simulink subsystem "NAV_GYRO_PROP"  (R2025b)
settings: Solver=VariableStepAuto  StartTime=0.0  StopTime=10.0  RelTol=1e-3
libraries: simulink x1
settings Model: Creator=antoniohernandez-rodiciomateos  LastModifiedBy=antoniohernandez-rodiciomateos

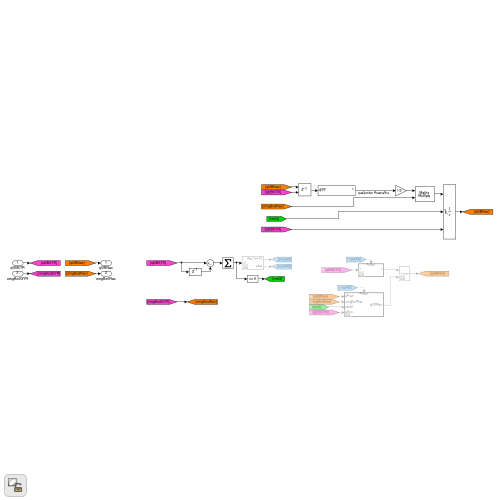
[thumbnail: Simulink's stored preview of the top-level diagram]
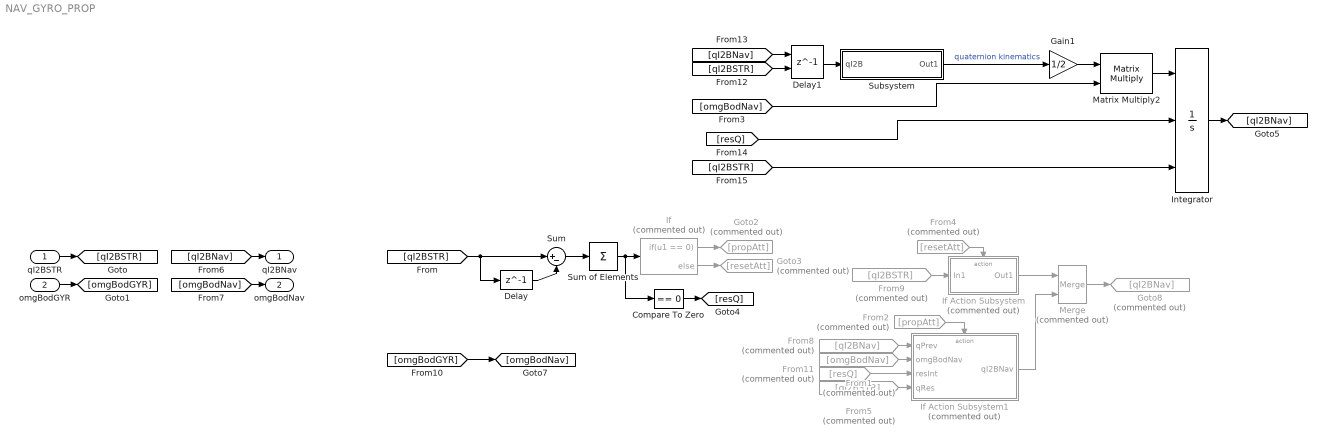
== system NAV_GYRO_PROP ==
  qI2BSTR : Inport  OutDataTypeStr=double  PortDimensions=[4 1]
  omgBodGYR : Inport  Port=2  OutDataTypeStr=double  PortDimensions=[3 1]
  Compare To Zero : simulink/Logic and Bit Operations/Compare To Zero  relop===  OutDataTypeStr=boolean
  Delay : Delay  DelayLength=1  InitialCondition=zeros(4, 1)
  Delay1 : Delay  DelayLength=1  InitialConditionSource=Input port
      settings: InputPortMap=u0,p4
  From1 : From  Commented=on  GotoTag=omgBodNav
  From11 : From  Commented=on  GotoTag=resQ
  From2 : From  Commented=on  GotoTag=propAtt
  From4 : From  Commented=on  GotoTag=resetAtt
  From5 : From  Commented=on  GotoTag=qI2BSTR
  From8 : From  Commented=on  GotoTag=qI2BNav
  From9 : From  Commented=on  GotoTag=qI2BSTR
  Gain1 : Gain  Gain=1/2
  Goto2 : Goto  Commented=on  GotoTag=propAtt
  Goto3 : Goto  Commented=on  GotoTag=resetAtt
  Goto8 : Goto  Commented=on  GotoTag=qI2BNav
  If : If  Commented=on  IfExpression=u1 == 0
  If Action Subsystem : Subsystem  Commented=on  TreatAsAtomicUnit=on
  If Action Subsystem1 : Subsystem  Commented=on  TreatAsAtomicUnit=on
  Integrator : Integrator  ExternalReset=falling  InitialConditionSource=external
  Matrix Multiply2 : Product  Multiplication=Matrix(*)
  Merge : Merge  Commented=on
  Subsystem : Subsystem
  Sum : Sum  Inputs=|+-
  Sum of Elements : Sum  Inputs=+
  qI2BNav : Outport  OutDataTypeStr=double  PortDimensions=[4 1]
  omgBodNav : Outport  Port=2  OutDataTypeStr=double  PortDimensions=[3 1]
  wires:
  qI2BSTR/1 -> [qI2BSTR]
  omgBodGYR/1 -> [omgBodGYR]
  [qI2BSTR] -> Sum/1, Delay/1
  Delay/1 -> Sum/2
  Sum/1 -> Sum of Elements/1
  Sum of Elements/1 -> If/1, Compare To Zero/1
  If/1 -> Goto2/1
  If/2 -> Goto3/1
  [qI2BNav] -> qI2BNav/1
  [omgBodNav] -> omgBodNav/1
  From4/1 -> If Action Subsystem/Action
  From9/1 -> If Action Subsystem/1(In1)
  [omgBodGYR] -> [omgBodNav]
  From1/1 -> If Action Subsystem1/2(omgBodNav)
  From11/1 -> If Action Subsystem1/3(resInt)
  From5/1 -> If Action Subsystem1/4(qRes)
  From8/1 -> If Action Subsystem1/1(qPrev)
  If Action Subsystem/1(Out1) -> Merge/1
  If Action Subsystem1/1(qI2BNav) -> Merge/2
  Merge/1 -> Goto8/1
  Compare To Zero/1 -> [resQ]
  From2/1 -> If Action Subsystem1/Action
  Matrix Multiply2/1 -> Integrator/1
  Subsystem/1(Out1) -> Gain1/1  "quaternion kinematics"
  Gain1/1 -> Matrix Multiply2/1
  Delay1/1 -> Subsystem/1(qI2B)
  Integrator/1 -> [qI2BNav]
  [qI2BSTR] -> Delay1/2
  [qI2BNav] -> Delay1/1
  [resQ] -> Integrator/2
  [omgBodNav] -> Matrix Multiply2/2
  [qI2BSTR] -> Integrator/3

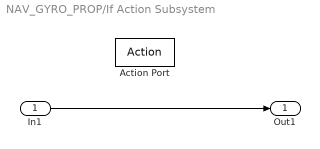
== system NAV_GYRO_PROP/If Action Subsystem ==
  In1 : Inport
  Action Port : ActionPort
  Out1 : Outport
  wires:
  In1/1 -> Out1/1

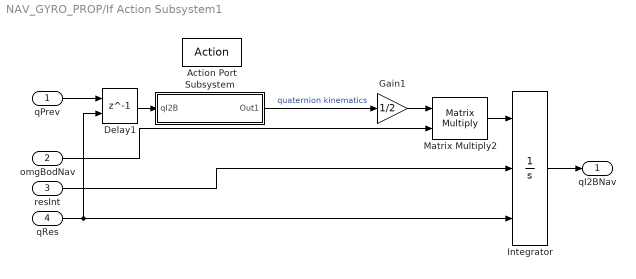
== system NAV_GYRO_PROP/If Action Subsystem1 ==
  qPrev : Inport  PortDimensions=[4 1]
  omgBodNav : Inport  Port=2  PortDimensions=[3 1]
  resInt : Inport  Port=3  PortDimensions=[1 1]
  qRes : Inport  Port=4  PortDimensions=[4 1]
  Action Port : ActionPort
  Delay1 : Delay  DelayLength=1  InitialConditionSource=Input port
      settings: InputPortMap=u0,p4
  Gain1 : Gain  Gain=1/2
  Integrator : Integrator  ExternalReset=falling  InitialConditionSource=external
  Matrix Multiply2 : Product  Multiplication=Matrix(*)
  Subsystem : Subsystem
  qI2BNav : Outport
  wires:
  Gain1/1 -> Matrix Multiply2/1
  qRes/1 -> Integrator/3, Delay1/2
  Subsystem/1(Out1) -> Gain1/1  "quaternion kinematics"
  resInt/1 -> Integrator/2
  Matrix Multiply2/1 -> Integrator/1
  omgBodNav/1 -> Matrix Multiply2/2
  Integrator/1 -> qI2BNav/1
  Delay1/1 -> Subsystem/1(qI2B)
  qPrev/1 -> Delay1/1

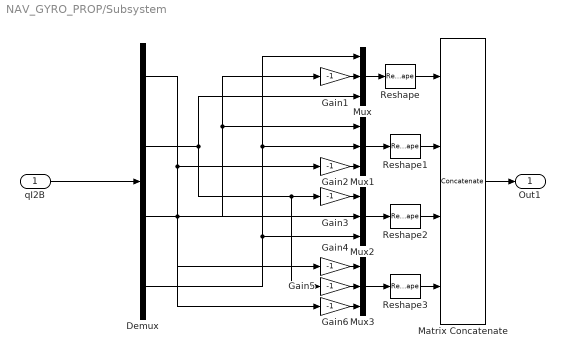
== system NAV_GYRO_PROP/Subsystem ==
  qI2B : Inport  PortDimensions=[4 1]
  Demux : Demux
  Gain{1..6} (6 alike) : Gain  Gain=-1
  Matrix Concatenate : Concatenate  NumInputs=4  Mode=Multidimensional array
  Mux{,1..3} (4 alike) : Mux  Inputs=3
  Reshape{,1..3} (4 alike) : Reshape  OutputDimensionality=Row vector (2-D)
  Out1 : Outport  PortDimensions=[4 3]
  wires:
  Demux/3 -> Gain1/1, Mux1/1, Gain6/1
  Reshape/1 -> Matrix Concatenate/1
  Demux/1 -> Gain2/1, Mux2/2, Gain4/1
  Gain6/1 -> Mux3/3
  Gain1/1 -> Mux/2
  Mux1/1 -> Reshape1/1
  Gain4/1 -> Mux3/1
  Demux/4 -> Mux/1, Mux1/2, Mux2/3
  Gain3/1 -> Mux2/1
  Demux/2 -> Mux/3, Gain3/1, Gain5/1
  Mux2/1 -> Reshape2/1
  Reshape3/1 -> Matrix Concatenate/4
  Gain5/1 -> Mux3/2
  Gain2/1 -> Mux1/3
  Reshape2/1 -> Matrix Concatenate/3
  Matrix Concatenate/1 -> Out1/1
  Mux3/1 -> Reshape3/1
  Reshape1/1 -> Matrix Concatenate/2
  Mux/1 -> Reshape/1
  qI2B/1 -> Demux/1

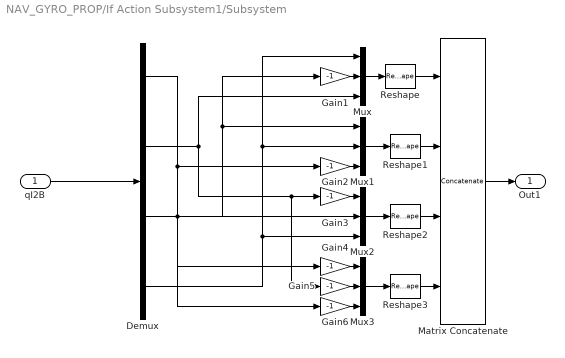
== system NAV_GYRO_PROP/If Action Subsystem1/Subsystem ==
  qI2B : Inport  PortDimensions=[4 1]
  Demux : Demux
  Gain{1..6} (6 alike) : Gain  Gain=-1
  Matrix Concatenate : Concatenate  NumInputs=4  Mode=Multidimensional array
  Mux{,1..3} (4 alike) : Mux  Inputs=3
  Reshape{,1..3} (4 alike) : Reshape  OutputDimensionality=Row vector (2-D)
  Out1 : Outport  PortDimensions=[4 3]
  wires:
  Demux/3 -> Gain1/1, Mux1/1, Gain6/1
  Reshape/1 -> Matrix Concatenate/1
  Demux/1 -> Gain2/1, Mux2/2, Gain4/1
  Gain6/1 -> Mux3/3
  Gain1/1 -> Mux/2
  Mux1/1 -> Reshape1/1
  Gain4/1 -> Mux3/1
  Demux/4 -> Mux/1, Mux1/2, Mux2/3
  Gain3/1 -> Mux2/1
  Demux/2 -> Mux/3, Gain3/1, Gain5/1
  Mux2/1 -> Reshape2/1
  Reshape3/1 -> Matrix Concatenate/4
  Gain5/1 -> Mux3/2
  Gain2/1 -> Mux1/3
  Reshape2/1 -> Matrix Concatenate/3
  Matrix Concatenate/1 -> Out1/1
  Mux3/1 -> Reshape3/1
  Reshape1/1 -> Matrix Concatenate/2
  Mux/1 -> Reshape/1
  qI2B/1 -> Demux/1
